simulink model "Model_Robust_14Bus_20pct"  (R2024b)
settings: Solver=FixedStepAuto  StartTime=0  StopTime=5  FixedStep=Ts  RelTol=1e-3
values from neighbouring files (symbols this model uses):
  ApparatusDiscreDamping =     [Data_Robust_14Bus_100pct.mat]    (also in Data_Robust_14Bus_20pct.mat; Data_Robust_14Bus_40pct.mat; Data_Robust_14Bus_60pct.mat; Data_Robust_14Bus_80pct.mat)
  ApparatusPara =     [Data_Robust_14Bus_100pct.mat]    (also in Data_Robust_14Bus_20pct.mat; Data_Robust_14Bus_40pct.mat; Data_Robust_14Bus_60pct.mat; Data_Robust_14Bus_80pct.mat)
  ApparatusPowerFlow =     [Data_Robust_14Bus_100pct.mat]    (also in Data_Robust_14Bus_20pct.mat; Data_Robust_14Bus_40pct.mat; Data_Robust_14Bus_60pct.mat; Data_Robust_14Bus_80pct.mat)
  ApparatusType =     [Data_Robust_14Bus_100pct.mat]    (also in Data_Robust_14Bus_20pct.mat; Data_Robust_14Bus_40pct.mat; Data_Robust_14Bus_60pct.mat; Data_Robust_14Bus_80pct.mat)
  Fbase = 60    [Data_Robust_14Bus_100pct.mat]    (also in Data_Robust_14Bus_20pct.mat; Data_Robust_14Bus_40pct.mat; Data_Robust_14Bus_60pct.mat; Data_Robust_14Bus_80pct.mat)
  OtherInputs =     [Data_Robust_14Bus_100pct.mat]    (also in Data_Robust_14Bus_20pct.mat; Data_Robust_14Bus_40pct.mat; Data_Robust_14Bus_60pct.mat; Data_Robust_14Bus_80pct.mat)
  Sbase = 1    [Data_Robust_14Bus_100pct.mat]    (also in Data_Robust_14Bus_20pct.mat; Data_Robust_14Bus_40pct.mat; Data_Robust_14Bus_60pct.mat; Data_Robust_14Bus_80pct.mat)
  Ts = 3.33333333333e-05    [Data_Robust_14Bus_100pct.mat]    (also in Data_Robust_14Bus_20pct.mat; Data_Robust_14Bus_40pct.mat; Data_Robust_14Bus_60pct.mat; Data_Robust_14Bus_80pct.mat)
  Vbase = 1    [Data_Robust_14Bus_100pct.mat]    (also in Data_Robust_14Bus_20pct.mat; Data_Robust_14Bus_40pct.mat; Data_Robust_14Bus_60pct.mat; Data_Robust_14Bus_80pct.mat)
  Wbase = 376.991118431    [Data_Robust_14Bus_100pct.mat]    (also in Data_Robust_14Bus_20pct.mat; Data_Robust_14Bus_40pct.mat; Data_Robust_14Bus_60pct.mat; Data_Robust_14Bus_80pct.mat)
  x_e =     [Data_Robust_14Bus_100pct.mat]    (also in Data_Robust_14Bus_20pct.mat; Data_Robust_14Bus_40pct.mat; Data_Robust_14Bus_60pct.mat; Data_Robust_14Bus_80pct.mat)
  Ybase = 1    [Data_Robust_14Bus_100pct.mat]    (also in Data_Robust_14Bus_20pct.mat; Data_Robust_14Bus_40pct.mat; Data_Robust_14Bus_60pct.mat; Data_Robust_14Bus_80pct.mat)
  Zbase = 1    [Data_Robust_14Bus_100pct.mat]    (also in Data_Robust_14Bus_20pct.mat; Data_Robust_14Bus_40pct.mat; Data_Robust_14Bus_60pct.mat; Data_Robust_14Bus_80pct.mat)
libraries: spsThreePhaseSeriesRLCBranchLib x20, SimplusGT x19, spsGroundLib x17, spsThreePhaseParallelRLCBranchLib x12, spsThreePhaseTransformerTwoWindingsLib x3, spspowerguiLib x1
settings Model: Creator=皮蛋蛋挞  LastModifiedBy=皮蛋蛋挞

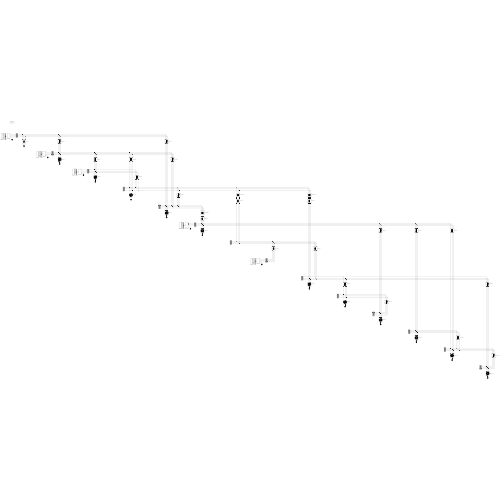
[thumbnail: Simulink's stored preview of the top-level diagram]
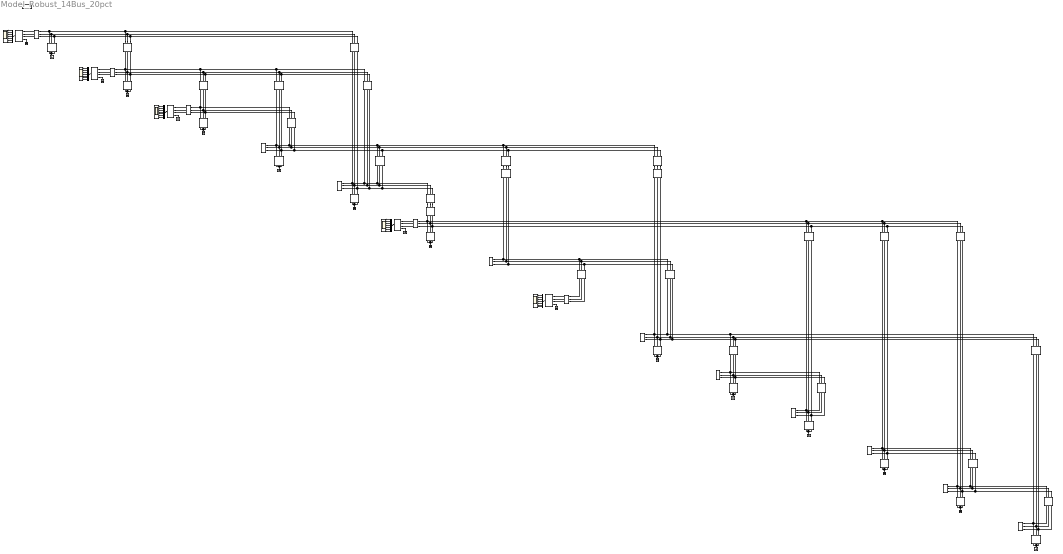
== system Model_Robust_14Bus_20pct ==
  B-GND{1,4,8,10,14,16,22,25,27..28,30,32} (12 alike) : spsGroundLib/Ground  LConnTagsString=a
  Branch1-1 : spsThreePhaseParallelRLCBranchLib/Three-Phase Parallel RLC Branch  LConnTagsString=A|B|C  RConnTagsString=A|B|C  BranchType=C  Resistance=(Inf)*Zbase  Inductance=(Inf)*Zbase/Wbase  Capacitance=(0.051)*Ybase/Wbase  Measurements=None
  Branch1-2 : spsThreePhaseSeriesRLCBranchLib/Three-Phase Series RLC Branch  LConnTagsString=A|B|C  RConnTagsString=A|B|C  BranchType=RL  Resistance=(0.01938)*Zbase  Inductance=(0.05917)*Zbase/Wbase  Capacitance=1e-6  Measurements=None
  Branch1-5 : spsThreePhaseSeriesRLCBranchLib/Three-Phase Series RLC Branch  LConnTagsString=A|B|C  RConnTagsString=A|B|C  BranchType=RL  Resistance=(0.05403)*Zbase  Inductance=(0.22304)*Zbase/Wbase  Capacitance=1e-6  Measurements=None
  Branch10-10 : spsThreePhaseParallelRLCBranchLib/Three-Phase Parallel RLC Branch  LConnTagsString=A|B|C  RConnTagsString=A|B|C  BranchType=RL  Resistance=(12.273)*Zbase  Inductance=(19.0443)*Zbase/Wbase  Capacitance=(0)*Ybase/Wbase  Measurements=None
  Branch10-11 : spsThreePhaseSeriesRLCBranchLib/Three-Phase Series RLC Branch  LConnTagsString=A|B|C  RConnTagsString=A|B|C  BranchType=RL  Resistance=(0.08205)*Zbase  Inductance=(0.19207)*Zbase/Wbase  Capacitance=1e-6  Measurements=None
  Branch11-11 : spsThreePhaseParallelRLCBranchLib/Three-Phase Parallel RLC Branch  LConnTagsString=A|B|C  RConnTagsString=A|B|C  BranchType=RL  Resistance=(31.9158)*Zbase  Inductance=(62.0584)*Zbase/Wbase  Capacitance=(0)*Ybase/Wbase  Measurements=None
  Branch12-12 : spsThreePhaseParallelRLCBranchLib/Three-Phase Parallel RLC Branch  LConnTagsString=A|B|C  RConnTagsString=A|B|C  BranchType=RL  Resistance=(18.2528)*Zbase  Inductance=(69.5889)*Zbase/Wbase  Capacitance=(0)*Ybase/Wbase  Measurements=None
  Branch12-13 : spsThreePhaseSeriesRLCBranchLib/Three-Phase Series RLC Branch  LConnTagsString=A|B|C  RConnTagsString=A|B|C  BranchType=RL  Resistance=(0.22092)*Zbase  Inductance=(0.19988)*Zbase/Wbase  Capacitance=1e-6  Measurements=None
  Branch13-13 : spsThreePhaseParallelRLCBranchLib/Three-Phase Parallel RLC Branch  LConnTagsString=A|B|C  RConnTagsString=A|B|C  BranchType=RL  Resistance=(8.1726)*Zbase  Inductance=(19.0224)*Zbase/Wbase  Capacitance=(0)*Ybase/Wbase  Measurements=None
  Branch13-14 : spsThreePhaseSeriesRLCBranchLib/Three-Phase Series RLC Branch  LConnTagsString=A|B|C  RConnTagsString=A|B|C  BranchType=RL  Resistance=(0.17093)*Zbase  Inductance=(0.34802)*Zbase/Wbase  Capacitance=1e-6  Measurements=None
  Branch14-14 : spsThreePhaseParallelRLCBranchLib/Three-Phase Parallel RLC Branch  LConnTagsString=A|B|C  RConnTagsString=A|B|C  BranchType=RL  Resistance=(7.1968)*Zbase  Inductance=(21.4464)*Zbase/Wbase  Capacitance=(0)*Ybase/Wbase  Measurements=None
  Branch2-2 : spsThreePhaseParallelRLCBranchLib/Three-Phase Parallel RLC Branch  LConnTagsString=A|B|C  RConnTagsString=A|B|C  BranchType=RLC  Resistance=(5.0324)*Zbase  Inductance=(8.5986)*Zbase/Wbase  Capacitance=(0.0826)*Ybase/Wbase  Measurements=None
  Branch2-3 : spsThreePhaseSeriesRLCBranchLib/Three-Phase Series RLC Branch  LConnTagsString=A|B|C  RConnTagsString=A|B|C  BranchType=RL  Resistance=(0.04699)*Zbase  Inductance=(0.19797)*Zbase/Wbase  Capacitance=1e-6  Measurements=None
  Branch2-4 : spsThreePhaseSeriesRLCBranchLib/Three-Phase Series RLC Branch  LConnTagsString=A|B|C  RConnTagsString=A|B|C  BranchType=RL  Resistance=(0.05811)*Zbase  Inductance=(0.17632)*Zbase/Wbase  Capacitance=1e-6  Measurements=None
  Branch2-5 : spsThreePhaseSeriesRLCBranchLib/Three-Phase Series RLC Branch  LConnTagsString=A|B|C  RConnTagsString=A|B|C  BranchType=RL  Resistance=(0.05695)*Zbase  Inductance=(0.17388)*Zbase/Wbase  Capacitance=1e-6  Measurements=None
  Branch3-3 : spsThreePhaseParallelRLCBranchLib/Three-Phase Parallel RLC Branch  LConnTagsString=A|B|C  RConnTagsString=A|B|C  BranchType=RLC  Resistance=(1.0829)*Zbase  Inductance=(5.3689)*Zbase/Wbase  Capacitance=(0.0283)*Ybase/Wbase  Measurements=None
  Branch3-4 : spsThreePhaseSeriesRLCBranchLib/Three-Phase Series RLC Branch  LConnTagsString=A|B|C  RConnTagsString=A|B|C  BranchType=RL  Resistance=(0.06701)*Zbase  Inductance=(0.17103)*Zbase/Wbase  Capacitance=1e-6  Measurements=None
  Branch4-4 : spsThreePhaseParallelRLCBranchLib/Three-Phase Parallel RLC Branch  LConnTagsString=A|B|C  RConnTagsString=A|B|C  BranchType=RC  Resistance=(2.1666)*Zbase  Inductance=(Inf)*Zbase/Wbase  Capacitance=(0.061057)*Ybase/Wbase  Measurements=None
  Branch4-5 : spsThreePhaseSeriesRLCBranchLib/Three-Phase Series RLC Branch  LConnTagsString=A|B|C  RConnTagsString=A|B|C  BranchType=RL  Resistance=(0.01335)*Zbase  Inductance=(0.04211)*Zbase/Wbase  Capacitance=1e-6  Measurements=None
  Branch4-7 : spsThreePhaseSeriesRLCBranchLib/Three-Phase Series RLC Branch  LConnTagsString=A|B|C  RConnTagsString=A|B|C  BranchType=L  Resistance=(0)*Zbase  Inductance=(0.20912)*Zbase/Wbase  Capacitance=1e-6  Measurements=None
  Branch4-9 : spsThreePhaseSeriesRLCBranchLib/Three-Phase Series RLC Branch  LConnTagsString=A|B|C  RConnTagsString=A|B|C  BranchType=L  Resistance=(0)*Zbase  Inductance=(0.55618)*Zbase/Wbase  Capacitance=1e-6  Measurements=None
  Branch5-5 : spsThreePhaseParallelRLCBranchLib/Three-Phase Parallel RLC Branch  LConnTagsString=A|B|C  RConnTagsString=A|B|C  BranchType=RLC  Resistance=(13.6764)*Zbase  Inductance=(64.963)*Zbase/Wbase  Capacitance=(0.0419)*Ybase/Wbase  Measurements=None
  Branch5-6 : spsThreePhaseSeriesRLCBranchLib/Three-Phase Series RLC Branch  LConnTagsString=A|B|C  RConnTagsString=A|B|C  BranchType=L  Resistance=(0)*Zbase  Inductance=(0.25202)*Zbase/Wbase  Capacitance=1e-6  Measurements=None
  Branch6-11 : spsThreePhaseSeriesRLCBranchLib/Three-Phase Series RLC Branch  LConnTagsString=A|B|C  RConnTagsString=A|B|C  BranchType=RL  Resistance=(0.09498)*Zbase  Inductance=(0.1989)*Zbase/Wbase  Capacitance=1e-6  Measurements=None
  Branch6-12 : spsThreePhaseSeriesRLCBranchLib/Three-Phase Series RLC Branch  LConnTagsString=A|B|C  RConnTagsString=A|B|C  BranchType=RL  Resistance=(0.12291)*Zbase  Inductance=(0.25581)*Zbase/Wbase  Capacitance=1e-6  Measurements=None
  Branch6-13 : spsThreePhaseSeriesRLCBranchLib/Three-Phase Series RLC Branch  LConnTagsString=A|B|C  RConnTagsString=A|B|C  BranchType=RL  Resistance=(0.06615)*Zbase  Inductance=(0.13027)*Zbase/Wbase  Capacitance=1e-6  Measurements=None
  Branch6-6 : spsThreePhaseParallelRLCBranchLib/Three-Phase Parallel RLC Branch  LConnTagsString=A|B|C  RConnTagsString=A|B|C  BranchType=RL  Resistance=(10.2223)*Zbase  Inductance=(15.2653)*Zbase/Wbase  Capacitance=(0)*Ybase/Wbase  Measurements=None
  Branch7-8 : spsThreePhaseSeriesRLCBranchLib/Three-Phase Series RLC Branch  LConnTagsString=A|B|C  RConnTagsString=A|B|C  BranchType=L  Resistance=(0)*Zbase  Inductance=(0.17615)*Zbase/Wbase  Capacitance=1e-6  Measurements=None
  Branch7-9 : spsThreePhaseSeriesRLCBranchLib/Three-Phase Series RLC Branch  LConnTagsString=A|B|C  RConnTagsString=A|B|C  BranchType=L  Resistance=(0)*Zbase  Inductance=(0.11001)*Zbase/Wbase  Capacitance=1e-6  Measurements=None
  Branch9-10 : spsThreePhaseSeriesRLCBranchLib/Three-Phase Series RLC Branch  LConnTagsString=A|B|C  RConnTagsString=A|B|C  BranchType=RL  Resistance=(0.03181)*Zbase  Inductance=(0.0845)*Zbase/Wbase  Capacitance=1e-6  Measurements=None
  Branch9-14 : spsThreePhaseSeriesRLCBranchLib/Three-Phase Series RLC Branch  LConnTagsString=A|B|C  RConnTagsString=A|B|C  BranchType=RL  Resistance=(0.12711)*Zbase  Inductance=(0.27038)*Zbase/Wbase  Capacitance=1e-6  Measurements=None
  Branch9-9 : spsThreePhaseParallelRLCBranchLib/Three-Phase Parallel RLC Branch  LConnTagsString=A|B|C  RConnTagsString=A|B|C  BranchType=RLC  Resistance=(3.7796)*Zbase  Inductance=(6.7168)*Zbase/Wbase  Capacitance=(0.19)*Ybase/Wbase  Measurements=None
  Bus{1..14} (14 alike) : SimplusGT/Three-Phase Bus  Vbase=1  Sbase=1
  D-GND{1..3,6,8} (5 alike) : spsGroundLib/Ground  LConnTagsString=a
  D-Scope{1..3,6,8} (5 alike) : Scope  NumInputPorts=7
  DS-Bus{1..3,6,8} (5 alike) : BusSelector  OutputSignals=v_dq,i_dq,v_abc,i_abc,w,theta,pq
  Transformer4-7 : spsThreePhaseTransformerTwoWindingsLib/Three-Phase Transformer (Two Windings)  Winding1Connection=Yg  Winding2Connection=Yg  CoreType=Three single-phase transformers  SetSaturation=off  Hysteresis=off  DataFile='hysteresis'  SetInitialFlux=off  Measurements=None  UNITS=pu  NominalPower=[Sbase, Fbase]  Winding1=[0.978*Vbase, 0, 0]  Winding2=[Vbase, 0, 0]  Rm=1e4  Lm=1e4  L0=0.5  Saturation=[ 0,0 ; 0.0024,1.2 ; 1.0,1.52 ]  InitialFluxes=[ 0.8 , -0.8 , 0.7 ]  BreakLoop=off  DiscreteSolver=Trapezoidal iterative  DataType=off  TransfoNumber=1
  Transformer4-9 : spsThreePhaseTransformerTwoWindingsLib/Three-Phase Transformer (Two Windings)  Winding1Connection=Yg  Winding2Connection=Yg  CoreType=Three single-phase transformers  SetSaturation=off  Hysteresis=off  DataFile='hysteresis'  SetInitialFlux=off  Measurements=None  UNITS=pu  NominalPower=[Sbase, Fbase]  Winding1=[0.969*Vbase, 0, 0]  Winding2=[Vbase, 0, 0]  Rm=1e4  Lm=1e4  L0=0.5  Saturation=[ 0,0 ; 0.0024,1.2 ; 1.0,1.52 ]  InitialFluxes=[ 0.8 , -0.8 , 0.7 ]  BreakLoop=off  DiscreteSolver=Trapezoidal iterative  DataType=off  TransfoNumber=1
  Transformer5-6 : spsThreePhaseTransformerTwoWindingsLib/Three-Phase Transformer (Two Windings)  Winding1Connection=Yg  Winding2Connection=Yg  CoreType=Three single-phase transformers  SetSaturation=off  Hysteresis=off  DataFile='hysteresis'  SetInitialFlux=off  Measurements=None  UNITS=pu  NominalPower=[Sbase, Fbase]  Winding1=[0.932*Vbase, 0, 0]  Winding2=[Vbase, 0, 0]  Rm=1e4  Lm=1e4  L0=0.5  Saturation=[ 0,0 ; 0.0024,1.2 ; 1.0,1.52 ]  InitialFluxes=[ 0.8 , -0.8 , 0.7 ]  BreakLoop=off  DiscreteSolver=Trapezoidal iterative  DataType=off  TransfoNumber=1
  VSI-Droop1 : SimplusGT/Grid-Forming Voltage-Source Inverter (dq-Frame System Object)  Ts=Ts  Sbase=Sbase  Vbase=Vbase  Wbase=Wbase  ApparatusType=ApparatusType{1}  ApparatusPara=ApparatusPara{1}  PowerFlow=ApparatusPowerFlow{1}  x0=x_e{1}  OtherInputs=OtherInputs{1}  DiscreMethod=Hybrid Trapezoidal  EnableInsideModification=off  DiscreDampingFlag=on  DiscreDampingValue=ApparatusDiscreDamping{1}  LinearizationTimes=1  DirectFeedthrough=off
  VSI-PLL2 : SimplusGT/Grid-Following Voltage-Source Inverter (dq-Frame System Object)  Ts=Ts  Sbase=Sbase  Vbase=Vbase  Wbase=Wbase  ApparatusType=ApparatusType{2}  ApparatusPara=ApparatusPara{2}  PowerFlow=ApparatusPowerFlow{2}  x0=x_e{2}  OtherInputs=OtherInputs{2}  DiscreMethod=Hybrid Trapezoidal  EnableInsideModification=off  DiscreDampingFlag=on  DiscreDampingValue=ApparatusDiscreDamping{2}  LinearizationTimes=1  DirectFeedthrough=off
  VSI-PLL3 : SimplusGT/Grid-Following Voltage-Source Inverter (dq-Frame System Object)  Ts=Ts  Sbase=Sbase  Vbase=Vbase  Wbase=Wbase  ApparatusType=ApparatusType{3}  ApparatusPara=ApparatusPara{3}  PowerFlow=ApparatusPowerFlow{3}  x0=x_e{3}  OtherInputs=OtherInputs{3}  DiscreMethod=Hybrid Trapezoidal  EnableInsideModification=off  DiscreDampingFlag=on  DiscreDampingValue=ApparatusDiscreDamping{3}  LinearizationTimes=1  DirectFeedthrough=off
  VSI-PLL6 : SimplusGT/Grid-Following Voltage-Source Inverter (dq-Frame System Object)  Ts=Ts  Sbase=Sbase  Vbase=Vbase  Wbase=Wbase  ApparatusType=ApparatusType{6}  ApparatusPara=ApparatusPara{6}  PowerFlow=ApparatusPowerFlow{6}  x0=x_e{6}  OtherInputs=OtherInputs{6}  DiscreMethod=Hybrid Trapezoidal  EnableInsideModification=off  DiscreDampingFlag=on  DiscreDampingValue=ApparatusDiscreDamping{6}  LinearizationTimes=1  DirectFeedthrough=off
  VSI-PLL8 : SimplusGT/Grid-Following Voltage-Source Inverter (dq-Frame System Object)  Ts=Ts  Sbase=Sbase  Vbase=Vbase  Wbase=Wbase  ApparatusType=ApparatusType{8}  ApparatusPara=ApparatusPara{8}  PowerFlow=ApparatusPowerFlow{8}  x0=x_e{8}  OtherInputs=OtherInputs{8}  DiscreMethod=Hybrid Trapezoidal  EnableInsideModification=off  DiscreDampingFlag=on  DiscreDampingValue=ApparatusDiscreDamping{8}  LinearizationTimes=1  DirectFeedthrough=off
  powergui : spspowerguiLib/powergui  Priority=1  SimulationMode=Discrete  SampleTime=Ts  frequency=60  Iterations=50  frequencyindice=60  Pbase=100e6  ErrMax=1e-4  UnitsV=kV  UnitsW=MW  buscounter=0  FunctionMessages=off  echomessages=off  EnableUseOfTLC=off  CurrentSourceSwitches=off  DisableSnubberDevices=off  DisableRonSwitches=off  DisableVfSwitches=off  DisplayEquations=off  AutomaticDiscreteSolvers=off  SolverType=Tustin/Backward Euler (TBE)  Interpol=off  ExternalGateDelay=off  methode=off  Ts=100  x0status=blocks  SPID=on  SwTol=0  HookPort=off  NonlinearTolerance=1e-4  nMaxIteration=100  ContinueOnMaxIteration=off  RestoreLinks=warning  ResistiveCurrentMeasurement=off  Frange=[0:2:500]  Ylog=off  Xlog=on  ShowGrid=off  save=off  variable=ZData  structure=0  ZoomFFT=off  StartTime=0.0  cycles=1  DisplayStyle=1  fundamental=60  FreqAxis=off  MaxFrequency=1000  frequencyindicesteady=1  RmsSteady=1  display=off
  wires:
  VSI-Droop1/1 -> DS-Bus1/1
  DS-Bus1/1 -> D-Scope1/1  "<v_dq>"
  DS-Bus1/2 -> D-Scope1/2  "<i_dq>"
  DS-Bus1/3 -> D-Scope1/3  "<v_abc>"
  DS-Bus1/4 -> D-Scope1/4  "<i_abc>"
  DS-Bus1/5 -> D-Scope1/5  "<w>"
  DS-Bus1/6 -> D-Scope1/6  "<theta>"
  DS-Bus1/7 -> D-Scope1/7  "<pq>"
  VSI-PLL2/1 -> DS-Bus2/1
  DS-Bus2/1 -> D-Scope2/1  "<v_dq>"
  DS-Bus2/2 -> D-Scope2/2  "<i_dq>"
  DS-Bus2/3 -> D-Scope2/3  "<v_abc>"
  DS-Bus2/4 -> D-Scope2/4  "<i_abc>"
  DS-Bus2/5 -> D-Scope2/5  "<w>"
  DS-Bus2/6 -> D-Scope2/6  "<theta>"
  DS-Bus2/7 -> D-Scope2/7  "<pq>"
  VSI-PLL3/1 -> DS-Bus3/1
  DS-Bus3/1 -> D-Scope3/1  "<v_dq>"
  DS-Bus3/2 -> D-Scope3/2  "<i_dq>"
  DS-Bus3/3 -> D-Scope3/3  "<v_abc>"
  DS-Bus3/4 -> D-Scope3/4  "<i_abc>"
  DS-Bus3/5 -> D-Scope3/5  "<w>"
  DS-Bus3/6 -> D-Scope3/6  "<theta>"
  DS-Bus3/7 -> D-Scope3/7  "<pq>"
  VSI-PLL6/1 -> DS-Bus6/1
  DS-Bus6/1 -> D-Scope6/1  "<v_dq>"
  DS-Bus6/2 -> D-Scope6/2  "<i_dq>"
  DS-Bus6/3 -> D-Scope6/3  "<v_abc>"
  DS-Bus6/4 -> D-Scope6/4  "<i_abc>"
  DS-Bus6/5 -> D-Scope6/5  "<w>"
  DS-Bus6/6 -> D-Scope6/6  "<theta>"
  DS-Bus6/7 -> D-Scope6/7  "<pq>"
  VSI-PLL8/1 -> DS-Bus8/1
  DS-Bus8/1 -> D-Scope8/1  "<v_dq>"
  DS-Bus8/2 -> D-Scope8/2  "<i_dq>"
  DS-Bus8/3 -> D-Scope8/3  "<v_abc>"
  DS-Bus8/4 -> D-Scope8/4  "<i_abc>"
  DS-Bus8/5 -> D-Scope8/5  "<w>"
  DS-Bus8/6 -> D-Scope8/6  "<theta>"
  DS-Bus8/7 -> D-Scope8/7  "<pq>"
  connections:
  VSI-Droop1/LConn4 -- D-GND1/LConn1
  VSI-PLL2/LConn4 -- D-GND2/LConn1
  VSI-PLL3/LConn4 -- D-GND3/LConn1
  VSI-PLL6/LConn4 -- D-GND6/LConn1
  VSI-PLL8/LConn4 -- D-GND8/LConn1
  Branch1-1/RConn1 -- Branch1-1/RConn2 -- Branch1-1/RConn3 -- B-GND1/LConn1
  Branch2-2/RConn1 -- Branch2-2/RConn2 -- Branch2-2/RConn3 -- B-GND4/LConn1
  Branch3-3/RConn1 -- Branch3-3/RConn2 -- Branch3-3/RConn3 -- B-GND8/LConn1
  Branch4-4/RConn1 -- Branch4-4/RConn2 -- Branch4-4/RConn3 -- B-GND10/LConn1
  Branch5-5/RConn1 -- Branch5-5/RConn2 -- Branch5-5/RConn3 -- B-GND14/LConn1
  Branch6-6/RConn1 -- Branch6-6/RConn2 -- Branch6-6/RConn3 -- B-GND16/LConn1
  Branch9-9/RConn1 -- Branch9-9/RConn2 -- Branch9-9/RConn3 -- B-GND22/LConn1
  Branch10-10/RConn1 -- Branch10-10/RConn2 -- Branch10-10/RConn3 -- B-GND25/LConn1
  Branch11-11/RConn1 -- Branch11-11/RConn2 -- Branch11-11/RConn3 -- B-GND27/LConn1
  Branch12-12/RConn1 -- Branch12-12/RConn2 -- Branch12-12/RConn3 -- B-GND28/LConn1
  Branch13-13/RConn1 -- Branch13-13/RConn2 -- Branch13-13/RConn3 -- B-GND30/LConn1
  Branch14-14/RConn1 -- Branch14-14/RConn2 -- Branch14-14/RConn3 -- B-GND32/LConn1
  Branch1-2/RConn1 -- Bus2/RConn1 -- Branch2-2/LConn1 -- Branch2-5/LConn1 -- Branch2-4/LConn1 -- Branch2-3/LConn1
  Branch1-2/RConn2 -- Bus2/RConn2 -- Branch2-2/LConn2 -- Branch2-5/LConn2 -- Branch2-4/LConn2 -- Branch2-3/LConn2
  Branch1-2/RConn3 -- Bus2/RConn3 -- Branch2-2/LConn3 -- Branch2-5/LConn3 -- Branch2-4/LConn3 -- Branch2-3/LConn3
  Branch1-2/LConn1 -- Bus1/RConn1 -- Branch1-1/LConn1 -- Branch1-5/LConn1
  Branch1-2/LConn2 -- Bus1/RConn2 -- Branch1-1/LConn2 -- Branch1-5/LConn2
  Branch1-2/LConn3 -- Bus1/RConn3 -- Branch1-1/LConn3 -- Branch1-5/LConn3
  Branch1-5/RConn1 -- Bus5/RConn1 -- Branch5-5/LConn1 -- Transformer5-6/LConn1 -- Branch4-5/RConn1 -- Branch2-5/RConn1
  Branch1-5/RConn2 -- Bus5/RConn2 -- Branch5-5/LConn2 -- Transformer5-6/LConn2 -- Branch4-5/RConn2 -- Branch2-5/RConn2
  Branch1-5/RConn3 -- Bus5/RConn3 -- Branch5-5/LConn3 -- Transformer5-6/LConn3 -- Branch4-5/RConn3 -- Branch2-5/RConn3
  Branch2-3/RConn1 -- Bus3/RConn1 -- Branch3-3/LConn1 -- Branch3-4/LConn1
  Branch2-3/RConn2 -- Bus3/RConn2 -- Branch3-3/LConn2 -- Branch3-4/LConn2
  Branch2-3/RConn3 -- Bus3/RConn3 -- Branch3-3/LConn3 -- Branch3-4/LConn3
  Branch2-4/RConn1 -- Bus4/RConn1 -- Branch4-4/LConn1 -- Transformer4-9/LConn1 -- Transformer4-7/LConn1 -- Branch4-5/LConn1 -- Branch3-4/RConn1
  Branch2-4/RConn2 -- Bus4/RConn2 -- Branch4-4/LConn2 -- Transformer4-9/LConn2 -- Transformer4-7/LConn2 -- Branch4-5/LConn2 -- Branch3-4/RConn2
  Branch2-4/RConn3 -- Bus4/RConn3 -- Branch4-4/LConn3 -- Transformer4-9/LConn3 -- Transformer4-7/LConn3 -- Branch4-5/LConn3 -- Branch3-4/RConn3
  Branch4-7/RConn1 -- Bus7/RConn1 -- Branch7-9/LConn1 -- Branch7-8/LConn1
  Branch4-7/RConn2 -- Bus7/RConn2 -- Branch7-9/LConn2 -- Branch7-8/LConn2
  Branch4-7/RConn3 -- Bus7/RConn3 -- Branch7-9/LConn3 -- Branch7-8/LConn3
  Transformer4-7/RConn1 -- Branch4-7/LConn1
  Transformer4-7/RConn2 -- Branch4-7/LConn2
  Transformer4-7/RConn3 -- Branch4-7/LConn3
  Branch4-9/RConn1 -- Bus9/RConn1 -- Branch9-9/LConn1 -- Branch9-14/LConn1 -- Branch9-10/LConn1 -- Branch7-9/RConn1
  Branch4-9/RConn2 -- Bus9/RConn2 -- Branch9-9/LConn2 -- Branch9-14/LConn2 -- Branch9-10/LConn2 -- Branch7-9/RConn2
  Branch4-9/RConn3 -- Bus9/RConn3 -- Branch9-9/LConn3 -- Branch9-14/LConn3 -- Branch9-10/LConn3 -- Branch7-9/RConn3
  Transformer4-9/RConn1 -- Branch4-9/LConn1
  Transformer4-9/RConn2 -- Branch4-9/LConn2
  Transformer4-9/RConn3 -- Branch4-9/LConn3
  Branch5-6/RConn1 -- Bus6/RConn1 -- Branch6-6/LConn1 -- Branch6-13/LConn1 -- Branch6-12/LConn1 -- Branch6-11/LConn1
  Branch5-6/RConn2 -- Bus6/RConn2 -- Branch6-6/LConn2 -- Branch6-13/LConn2 -- Branch6-12/LConn2 -- Branch6-11/LConn2
  Branch5-6/RConn3 -- Bus6/RConn3 -- Branch6-6/LConn3 -- Branch6-13/LConn3 -- Branch6-12/LConn3 -- Branch6-11/LConn3
  Transformer5-6/RConn1 -- Branch5-6/LConn1
  Transformer5-6/RConn2 -- Branch5-6/LConn2
  Transformer5-6/RConn3 -- Branch5-6/LConn3
  Branch6-11/RConn1 -- Bus11/RConn1 -- Branch11-11/LConn1 -- Branch10-11/RConn1
  Branch6-11/RConn2 -- Bus11/RConn2 -- Branch11-11/LConn2 -- Branch10-11/RConn2
  Branch6-11/RConn3 -- Bus11/RConn3 -- Branch11-11/LConn3 -- Branch10-11/RConn3
  Branch6-12/RConn1 -- Bus12/RConn1 -- Branch12-12/LConn1 -- Branch12-13/LConn1
  Branch6-12/RConn2 -- Bus12/RConn2 -- Branch12-12/LConn2 -- Branch12-13/LConn2
  Branch6-12/RConn3 -- Bus12/RConn3 -- Branch12-12/LConn3 -- Branch12-13/LConn3
  Branch6-13/RConn1 -- Bus13/RConn1 -- Branch13-13/LConn1 -- Branch13-14/LConn1 -- Branch12-13/RConn1
  Branch6-13/RConn2 -- Bus13/RConn2 -- Branch13-13/LConn2 -- Branch13-14/LConn2 -- Branch12-13/RConn2
  Branch6-13/RConn3 -- Bus13/RConn3 -- Branch13-13/LConn3 -- Branch13-14/LConn3 -- Branch12-13/RConn3
  Bus8/RConn1 -- Branch7-8/RConn1
  Bus8/RConn2 -- Branch7-8/RConn2
  Bus8/RConn3 -- Branch7-8/RConn3
  Branch9-10/RConn1 -- Bus10/RConn1 -- Branch10-10/LConn1 -- Branch10-11/LConn1
  Branch9-10/RConn2 -- Bus10/RConn2 -- Branch10-10/LConn2 -- Branch10-11/LConn2
  Branch9-10/RConn3 -- Bus10/RConn3 -- Branch10-10/LConn3 -- Branch10-11/LConn3
  Branch9-14/RConn1 -- Bus14/RConn1 -- Branch14-14/LConn1 -- Branch13-14/RConn1
  Branch9-14/RConn2 -- Bus14/RConn2 -- Branch14-14/LConn2 -- Branch13-14/RConn2
  Branch9-14/RConn3 -- Bus14/RConn3 -- Branch14-14/LConn3 -- Branch13-14/RConn3
  VSI-Droop1/LConn1 -- Bus1/LConn1
  VSI-Droop1/LConn2 -- Bus1/LConn2
  VSI-Droop1/LConn3 -- Bus1/LConn3
  VSI-PLL2/LConn1 -- Bus2/LConn1
  VSI-PLL2/LConn2 -- Bus2/LConn2
  VSI-PLL2/LConn3 -- Bus2/LConn3
  VSI-PLL3/LConn1 -- Bus3/LConn1
  VSI-PLL3/LConn2 -- Bus3/LConn2
  VSI-PLL3/LConn3 -- Bus3/LConn3
  VSI-PLL6/LConn1 -- Bus6/LConn1
  VSI-PLL6/LConn2 -- Bus6/LConn2
  VSI-PLL6/LConn3 -- Bus6/LConn3
  VSI-PLL8/LConn1 -- Bus8/LConn1
  VSI-PLL8/LConn2 -- Bus8/LConn2
  VSI-PLL8/LConn3 -- Bus8/LConn3
